simulink model "Golf_Nonlin_Optimale"  (R2019a)
settings: Solver=VariableStepAuto  StartTime=0.0  StopTime=1000  RelTol=1e-3
values from neighbouring files (symbols this model uses):
  DEG2RAD = pi/180.    (= 0.0174532925199)    [mainProjetCADV_2a.m]    (also in utAcDynamicsFunction.m; utConstantAeroCoeff.m)
  km = trim.kmass(choix)    [utGetTrimPoint.m]
  KTS2MS = 1852 / 3600    (= 0.514444444444)    [mainProjetCADV_2a.m]    (also in utAcDynamicsFunction.m)
  ms = trim.mStat(choix)    [utGetTrimPoint.m]
  xTrim = zeros(TOTAL_SV, 1)    [mainProjetCADV_2a.m]
undefined symbols (not defined in the file or in its folder): aircraftChosen, alphaTrimLF, Ar, Br, C_sys, Cr, Dpf, dPHRTrimLF, Dr, dthrTrimLF, Kr, Kx, thetaTrimLF, VaTrimLF
settings Model: Creator=mariu  LastModifiedBy=ulyss

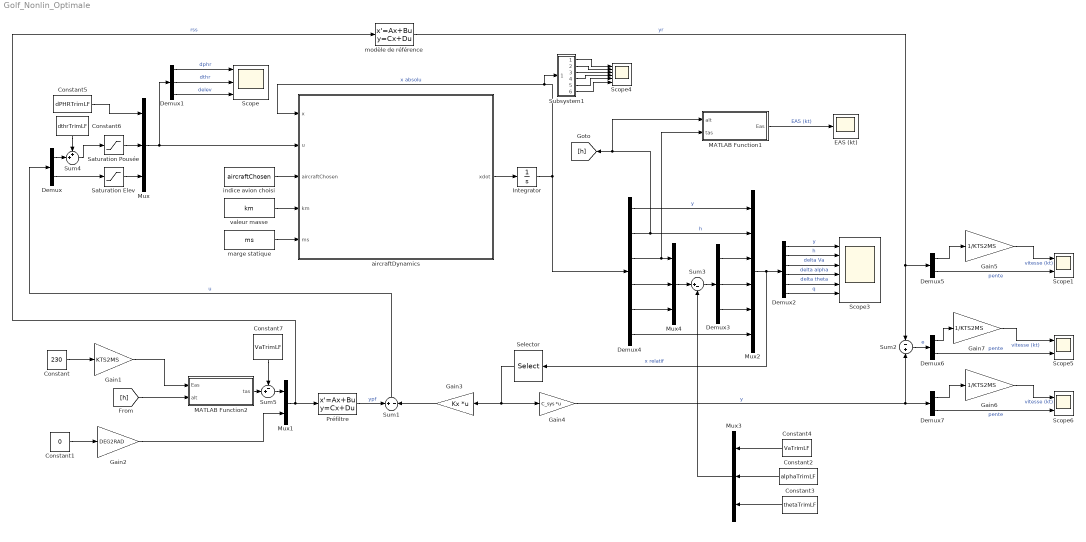
== system Golf_Nonlin_Optimale ==
  Constant : Constant  Value=230
  Constant1 : Constant  Value=0
  Constant2 : Constant  Value=alphaTrimLF
  Constant3 : Constant  Value=thetaTrimLF
  Constant4 : Constant  Value=VaTrimLF
  Constant5 : Constant  Value=dPHRTrimLF
  Constant6 : Constant  Value=dthrTrimLF
  Constant7 : Constant  Value=VaTrimLF
  Demux{,5..7} (4 alike) : Demux  Outputs=2
  Demux1 : Demux  Outputs=3
  Demux2 : Demux  Outputs=6
  Demux3 : Demux  Outputs=3
  Demux4 : Demux  Outputs=6
  EAS (kt) : Scope
  Gain1 : Gain  Gain=KTS2MS
  Gain2 : Gain  Gain=DEG2RAD
  Gain3 : Gain  Gain=Kx  Multiplication=Matrix(K*u) (u vector)
  Gain4 : Gain  Gain=C_sys  Multiplication=Matrix(K*u) (u vector)
  Gain5 : Gain  Gain=1/KTS2MS
  Gain6 : Gain  Gain=1/KTS2MS
  Gain7 : Gain  Gain=1/KTS2MS
  Integrator : Integrator  InitialCondition=xTrim
  MATLAB Function1 : MATLAB Function  TreatAsAtomicUnit=on
  MATLAB Function2 : MATLAB Function  TreatAsAtomicUnit=on
  Mux : Mux  Inputs=3
  Mux1 : Mux  Inputs=2
  Mux2 : Mux  Inputs=6
  Mux3 : Mux  Inputs=3
  Mux4 : Mux  Inputs=3
  Préfiltre : StateSpace  A=Ar  B=Br  C=-Kr  D=Dpf  InitialCondition=0
  Saturation Elev : Saturate  UpperLimit=30*DEG2RAD  LowerLimit=-30*DEG2RAD
  Saturation Pousée : Saturate  UpperLimit=1  LowerLimit=0
  Scope : Scope  NumInputPorts=3
  Scope1 : Scope  NumInputPorts=2
  Scope3 : Scope  NumInputPorts=6
  Scope4 : Scope  NumInputPorts=6
  Scope5 : Scope  NumInputPorts=2
  Scope6 : Scope  NumInputPorts=2
  Selector : Selector  InputPortWidth=6  IndexOptions=Index vector (dialog)  Indices=[3:6]  OutputSizes=1
  Subsystem1 : Subsystem
  Sum1 : Sum  Inputs=+|-
  Sum2 : Sum  Inputs=-|+
  Sum3 : Sum  Inputs=|+-
  Sum4 : Sum  Inputs=++|
  Sum5 : Sum  Inputs=-+|
  aircraftDynamics : MATLAB Function  TreatAsAtomicUnit=on
  indice avion choisi : Constant  Value=aircraftChosen
  marge statique : Constant  Value=ms
  modèle de référence : StateSpace  A=Ar  B=Br  C=Cr  D=Dr  InitialCondition=0
  valeur masse : Constant  Value=km
  wires:
  marge statique/1 -> aircraftDynamics/5(ms)
  aircraftDynamics/1(xdot) -> Integrator/1
  indice avion choisi/1 -> aircraftDynamics/3(aircraftChosen)
  valeur masse/1 -> aircraftDynamics/4(km)
  Gain3/1 -> Sum1/2
  Sum1/1 -> Demux/1  "u"
  Constant1/1 -> Gain2/1
  Gain1/1 -> MATLAB Function2/1(Eas)
  Constant/1 -> Gain1/1
  Gain2/1 -> Mux1/2
  Préfiltre/1 -> Sum1/1  "ypf"
  Mux1/1 -> Préfiltre/1, modèle de référence/1  "rss"
  modèle de référence/1 -> Sum2/1, Demux5/1  "yr"
  Selector/1 -> Gain3/1, Gain4/1
  Mux/1 -> aircraftDynamics/2(u), Demux1/1
  Integrator/1 -> aircraftDynamics/1(x), Subsystem1/1(In1), Demux4/1  "x absolu"
  Demux2/3 -> Scope3/3  "delta Va"
  Mux2/1 -> Selector/1, Demux2/1  "x relatif"
  Demux2/6 -> Scope3/6  "q"
  MATLAB Function1/1(Eas) -> EAS (kt)/1  "EAS (kt)"
  Sum3/1 -> Demux3/1
  Demux2/4 -> Scope3/4  "delta alpha"
  Demux2/5 -> Scope3/5  "delta theta"
  Mux4/1 -> Sum3/1
  Constant5/1 -> Mux/1
  Subsystem1/1(delta Va) -> Scope4/1
  Subsystem1/2(delta alpha) -> Scope4/2
  Subsystem1/3(delta theta) -> Scope4/3
  Subsystem1/4(delta q) -> Scope4/4
  Subsystem1/5(etat pid) -> Scope4/5
  Subsystem1/6(etat pf) -> Scope4/6
  Demux/1 -> Sum4/2
  Constant6/1 -> Sum4/1
  Demux2/2 -> Scope3/2  "h"
  Demux2/1 -> Scope3/1  "y"
  Mux3/1 -> Sum3/2
  Constant4/1 -> Mux3/1
  Constant2/1 -> Mux3/2
  Constant3/1 -> Mux3/3
  Demux4/5 -> Mux4/3
  Demux4/4 -> Mux4/2
  Demux4/3 -> MATLAB Function1/2(tas), Mux4/1
  Demux3/1 -> Mux2/3
  Demux3/2 -> Mux2/4
  Demux3/3 -> Mux2/5
  Demux4/6 -> Mux2/6
  Demux4/2 -> MATLAB Function1/1(alt), [h], Mux2/2  "h"
  Demux4/1 -> Mux2/1  "y"
  [h] -> MATLAB Function2/2(alt)
  Demux5/1 -> Gain5/1
  Demux5/2 -> Scope1/2  "pente"
  Gain4/1 -> Sum2/2, Demux7/1  "y"
  Gain5/1 -> Scope1/1  "vitesse (kt)"
  Demux7/2 -> Scope6/2  "pente"
  Gain6/1 -> Scope6/1  "vitesse (kt)"
  Demux7/1 -> Gain6/1
  MATLAB Function2/1(tas) -> Sum5/2
  Sum5/1 -> Mux1/1
  Constant7/1 -> Sum5/1
  Demux6/2 -> Scope5/2  "pente"
  Gain7/1 -> Scope5/1  "vitesse (kt)"
  Demux6/1 -> Gain7/1
  Sum2/1 -> Demux6/1  "e"
  Demux1/1 -> Scope/1  "dphr"
  Demux1/2 -> Scope/2  "dthr"
  Saturation Pousée/1 -> Mux/2
  Sum4/1 -> Saturation Pousée/1
  Demux1/3 -> Scope/3  "delev"
  Saturation Elev/1 -> Mux/3
  Demux/2 -> Saturation Elev/1

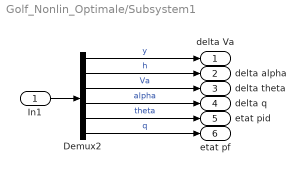
== system Golf_Nonlin_Optimale/Subsystem1 ==
  In1 : Inport
  Demux2 : Demux  Outputs=6
  delta Va : Outport
  delta alpha : Outport  Port=2
  delta theta : Outport  Port=3
  delta q : Outport  Port=4
  etat pid : Outport  Port=5
  etat pf : Outport  Port=6
  wires:
  Demux2/3 -> delta theta/1  "Va"
  Demux2/1 -> delta Va/1  "y"
  Demux2/6 -> etat pf/1  "q"
  Demux2/5 -> etat pid/1  "theta"
  Demux2/2 -> delta alpha/1  "h"
  In1/1 -> Demux2/1
  Demux2/4 -> delta q/1  "alpha"

== matlab function Golf_Nonlin_Optimale/MATLAB Function2 ==
  data: Eas input; alt input; tas output
function tas = utEas2tas(Eas, alt)
    %tas, Eas (%equivalent vitesse) en m/s
    %alt en m
    %cf. http://www.hochwarth.com/misc/AviationCalculator.html
    tas = sqrt(utRho(0)/utRho(alt))*Eas;
end

== matlab function Golf_Nonlin_Optimale/aircraftDynamics ==
  data: x input; u input; xdot output; aircraftChosen input; km input; ms input
function xdot = aircraftDynamics(x,u, aircraftChosen,km,ms)
    TOTAL_SV = 6;
    xIn = zeros(TOTAL_SV,1);
    xIn = x;
    
	TOTAL_CMD = 3;
    uIn = zeros(TOTAL_CMD,1);
    uIn = u;
    
    xdot = utAcDynamicsFunction(xIn,uIn, aircraftChosen,km,ms);
end %aircraftDynamics

== matlab function Golf_Nonlin_Optimale/MATLAB Function1 ==
  data: alt input; tas input; Eas output
function Eas = utTas2Eas(alt, tas)
    %tas, Eas(%equivalent vitesse) en m/s
    %alt en m
    %cf. http://www.hochwarth.com/misc/AviationCalculator.html
    Eas = sqrt(utRho(alt)/utRho(0))*tas/0.5144;
    %sortie en kt
end
